simulink model "Environment"  (R2024a)
settings: Solver=ode15s  StartTime=0.0  StopTime=50  FixedStep=0.04  MaxStep=0.04  RelTol=1e-3
values from neighbouring files (symbols this model uses):
  h = 2.7    [Variabili.m]
  traiettoria = [x', y']    [generatoreTraiettoria.m]    (also in generatoreTraiettoria2.m; tra3.m)
  w = 1.4    [Variabili.m]
libraries: simulink x2, rllib x1
settings Model: Creator=Luzi  LastModifiedBy=francesco
settings RTWCC: GPUComputeCapability=3.5

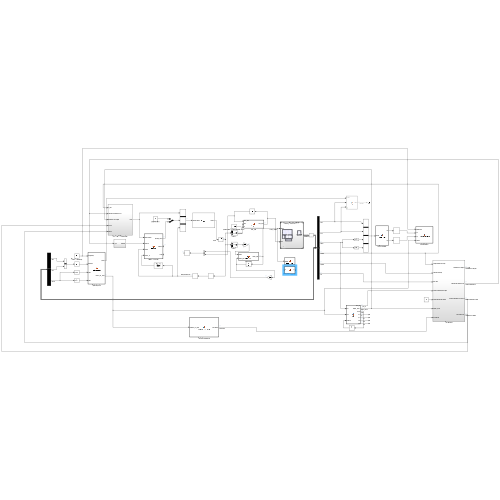
[thumbnail: Simulink's stored preview of the top-level diagram]
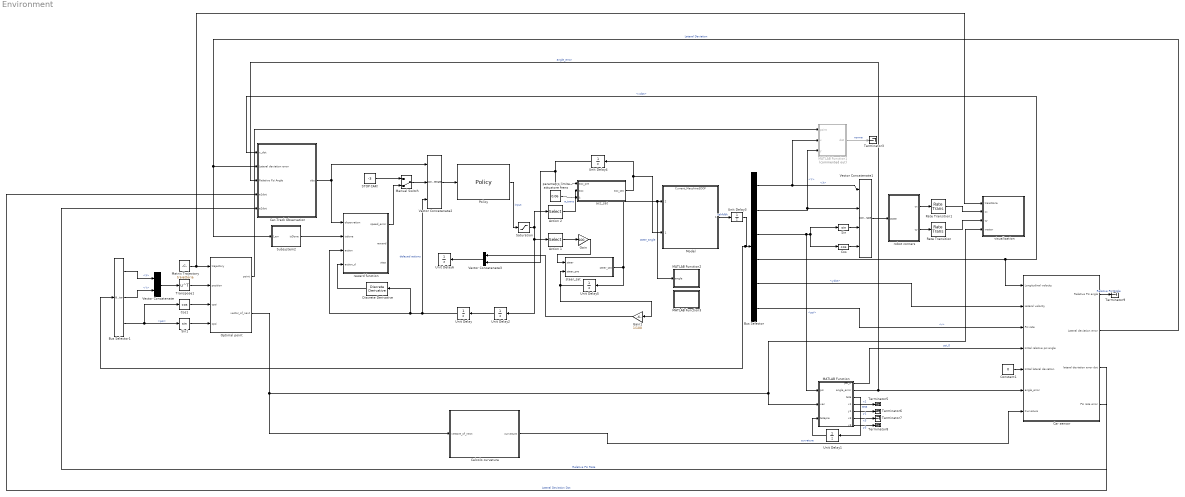
== system Environment ==
  Action 1 : Selector  InputPortWidth=2  IndexOptions=Index vector (dialog)  Indices=1  OutputSizes=1
  Action 2 : Selector  InputPortWidth=2  IndexOptions=Index vector (dialog)  Indices=2  OutputSizes=1
  Bus Selector : BusSelector  OutputSignals=InertFrm.Cg.Disp.X,InertFrm.Cg.Disp.Y,InertFrm.Cg.Ang.psi,BdyFrm.Cg.Vel.xdot,BdyFrm.Cg.Vel.ydot,BdyFrm.Cg.AngVel.r
  Bus Selector1 : BusSelector  OutputSignals=InertFrm.Cg.Disp.X,InertFrm.Cg.Disp.Y,InertFrm.Cg.Ang.psi
  Calcolo curvatura : MATLAB Function  TreatAsAtomicUnit=on
  Car sensor : Subsystem
  Car-Track Observation : Subsystem
  Constant1 : Constant  Value=0
  Cos : Trigonometry  Operator=cos
  Cos1 : Trigonometry  Operator=cos
  Discrete Derivative : simulink/Discrete/Discrete Derivative  gainval=0.1  ICPrevScaledInput=0.0  OutMin=[]  OutMax=[]  OutDataType=fixdt(1, 16)  OutScaling=2^-10  DoSatur=off
  Gain : Gain  Gain=100
  Gain1 : Gain  Gain=1/100
  MATLAB Function : MATLAB Function  TreatAsAtomicUnit=on
  MATLAB Function1 : MATLAB Function  Commented=on  TreatAsAtomicUnit=on
  MATLAB Function2 : MATLAB Function  TreatAsAtomicUnit=on
  MATLAB Function3 : MATLAB Function  TreatAsAtomicUnit=on
  Manual Switch : ManualSwitch  CurrentSetting=0
  Matrix Trajectory : Constant  Value=traiettoria  SampleTime=60
  Model : ModelReference  ModelNameDialog=Current_Macchina3DOF.slx  SimulationMode=Normal  ModelReferenceVersion=1.72
      settings: PortSchema="{\"entries\":[{\"content\":{\"sides\":[{\"content\":{\"connectorIds\":[\"In2\",\"In1\"]},\"type\":\"ConnectorPlacement.EquallySpacedRectSide\",\"uuid\":\"b5a44853-6584-4a50-847d-9a0b1c5ea9ac\"},{\"content\":{\"connectorIds\":[\"Out1\"],\"side\":\"RIGHT\"},\"type\":\"ConnectorPlacement.EquallySpacedRectSide\",\"uuid\":\"bfcb6c88-1d93-4f70-bf16-2c719fa247ba\"},{\"content\":{\"side\":\"TOP\"},\"type\":\"ConnectorPlacement.EquallySpacedRectSide\",\"uuid\":\"3385b00b-6ed4-40a5-8204-01acdd431cf5\"}]},\"type\":\"ConnectorPlacement.EquallySpacedConnector\",\"uuid\":\"3bb36942-6fbc-4d27-a33b-ca1de48b267b\"}],\"packageUris\":[\"http://schema.mathworks.com/mf0/Connector/R2020b\"],\"version\":\"1.0\"}"
  Optimal point : MATLAB Function  TreatAsAtomicUnit=on
  Policy : rllib/Policy  MATFile=/Users/francesco/Repository/FS/HL/High Level Control RL_Training/agentData25hz.mat  PolicyParamsAsInput=off  PolicyParamsBusName=policy_param_bus  SimUsingCodegen=off
  Rate Transition : RateTransition
  Rate Transition1 : RateTransition
  STOP CAR! : Constant  Value=-3
  Saturation : Saturate  UpperLimit=1  LowerLimit=-1
  Sin : Trigonometry
  Sin1 : Trigonometry
  Subsystem2 : Subsystem
  Terminator{3,5..9} (6 alike) : Terminator
  Transpose1 : Math  Operator=transpose
  Unit Delay{,1..6} (7 alike) : UnitDelay  SampleTime=-1  HasFrameUpgradeWarning=on
  Vector Concatenate : Concatenate
  Vector Concatenate1 : Concatenate  NumInputs=4
  Vector Concatenate2 : Concatenate  NumInputs=3
  Vector Concatenate3 : Concatenate
  acc_sat : MATLAB Function  TreatAsAtomicUnit=on
  parametro limite attuatore freno : Constant  Value=0.06
  reward function : MATLAB Function  TreatAsAtomicUnit=on
  robot corners : MATLAB Function  TreatAsAtomicUnit=on
  steer_sat : MATLAB Function  TreatAsAtomicUnit=on
  visualization : MATLAB Function  TreatAsAtomicUnit=on
  wires:
  Policy/1 -> Saturation/1  "input"
  Bus Selector/6 -> Car sensor/3(Psi rate)  "<r>"
  Bus Selector/4 -> Car sensor/1(Longitudinal velocity), Car-Track Observation/1(x_dot)  "<xdot>"
  Sin/1 -> Vector Concatenate1/3
  Cos/1 -> Vector Concatenate1/4
  Unit Delay2/1 -> Unit Delay/1
  Bus Selector1/1 -> Vector Concatenate/1  "<X>"
  Bus Selector1/2 -> Vector Concatenate/2  "<Y>"
  Matrix Trajectory/1 -> Optimal point/1(trajectory), visualization/1(traiettoria)
  Cos1/1 -> Optimal point/3(cpsi)
  Vector Concatenate/1 -> Transpose1/1
  Transpose1/1 -> Optimal point/2(position)
  robot corners/2(cy) -> Rate Transition/1
  robot corners/1(cx) -> Rate Transition1/1
  Unit Delay3/1 -> Bus Selector1/1, Bus Selector/1
  Bus Selector1/3 -> Cos1/1, Sin1/1  "<psi>"
  Sin1/1 -> Optimal point/4(spsi)
  Vector Concatenate1/1 -> robot corners/1(state)
  Bus Selector/5 -> Car sensor/2(Lateral velocity)  "<ydot>"
  Calcolo curvatura/1(curvatura) -> Car sensor/7(Curvature)  "curvature"
  MATLAB Function/1(psi_0) -> Car sensor/4(Initial relative psi angle)  "psi_0"
  Car sensor/3(lateral deviation error dot) -> Car-Track Observation/4(e1dot)  "Lateral Deviation Dot"
  Car sensor/4(Psi rate error) -> Car-Track Observation/5(e2dot)  "Relative Psi Rate"
  Car sensor/2(Lateral deviation error) -> Car-Track Observation/2(Lateral deviation error), Subsystem2/1(l_err)  "Lateral Deviation"
  Vector Concatenate2/1 -> Policy/1
  Car-Track Observation/1(obs) -> Vector Concatenate2/1, reward function/1(observation)
  Optimal point/1(point) -> MATLAB Function1/1(point)
  Optimal point/2(vector_of_next) -> Calcolo curvatura/1(vettore_of_next), visualization/4(vector), MATLAB Function/2(vec)
  Model/1 -> Unit Delay3/1  "vehfdbk"
  Rate Transition1/1 -> visualization/2(cx)
  Rate Transition/1 -> visualization/3(cy)
  Unit Delay/1 -> Vector Concatenate2/3, reward function/3(action), Discrete Derivative/1  "delayed actions"
  Saturation/1 -> Unit Delay2/1, Action 1/1, Action 2/1
  Discrete Derivative/1 -> reward function/4(action_d)
  Bus Selector/1 -> Vector Concatenate1/1, MATLAB Function1/2(x)  "<X>"
  Bus Selector/2 -> MATLAB Function1/3(y), Vector Concatenate1/2  "<Y>"
  Bus Selector/3 -> MATLAB Function/1(psi), Cos/1, Sin/1  "<psi>"
  MATLAB Function/2(angle_error) -> Car-Track Observation/3(Relative Psi Angle), Car sensor/6(angle_error)  "angle_error"
  MATLAB Function1/1(dist) -> Terminator3/1  "norma"
  MATLAB Function/3(teta) -> Unit Delay1/1  "teta"
  Constant1/1 -> Car sensor/5(Initial lateral deviation)
  MATLAB Function/4(x1) -> Terminator5/1  "x1"
  MATLAB Function/5(y1) -> Terminator6/1  "y1"
  MATLAB Function/6(x3) -> Terminator7/1  "x3"
  MATLAB Function/7(y3) -> Terminator8/1  "y3"
  Car sensor/1(Relative Psi angle) -> Terminator9/1  "Relative Psi Angle"
  Unit Delay1/1 -> MATLAB Function/3(tetapre)
  Unit Delay4/1 -> Vector Concatenate3/2, acc_sat/1(acc_pre)
  acc_sat/1(acc_sat) -> Unit Delay4/1, Model/1
  Unit Delay5/1 -> steer_sat/2(steer_pre), Gain1/1
  steer_sat/1(steer_sat) -> Unit Delay5/1, MATLAB Function2/1(angle), Model/2  "steer_angle"
  Action 1/1 -> Gain/1
  Subsystem2/1(isDone) -> reward function/2(isdone)
  Gain/1 -> steer_sat/1(steer)
  Vector Concatenate3/1 -> Unit Delay6/1
  Gain1/1 -> Vector Concatenate3/1
  reward function/1(speed_error) -> Manual Switch/2
  Manual Switch/1 -> Vector Concatenate2/2
  STOP CAR!/1 -> Manual Switch/1
  Action 2/1 -> acc_sat/2(acc)  "a_trans"
  parametro limite attuatore freno/1 -> acc_sat/3(k)

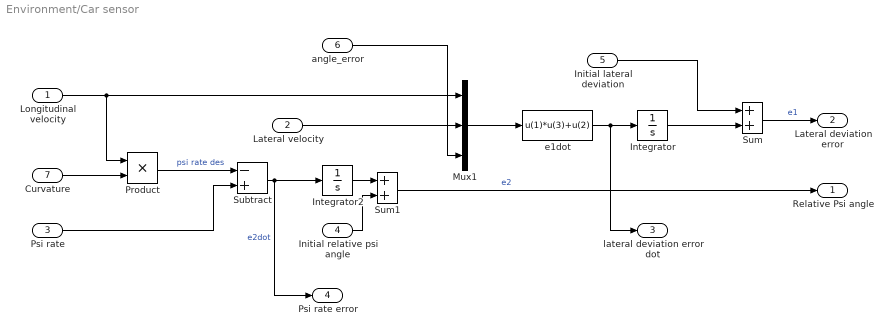
== system Environment/Car sensor ==
  Longitudinal velocity : Inport
  Lateral velocity : Inport  Port=2
  Psi rate : Inport  Port=3
  Initial relative psi angle : Inport  Port=4
  Initial lateral deviation : Inport  Port=5
  angle_error : Inport  Port=6
  Curvature : Inport  Port=7
  Integrator : Integrator
  Integrator2 : Integrator
  Mux1 : Mux  Inputs=[1 1 1]
  Product : Product
  Subtract : Sum  Inputs=-+
  Sum : Sum
  Sum1 : Sum
  e1dot : Fcn  Expr=u(1)*u(3)+u(2)
  Relative Psi angle : Outport  VectorParamsAs1DForOutWhenUnconnected=off
  Lateral deviation error : Outport  Port=2  VectorParamsAs1DForOutWhenUnconnected=off
  lateral deviation error dot : Outport  Port=3  VectorParamsAs1DForOutWhenUnconnected=off
  Psi rate error : Outport  Port=4  VectorParamsAs1DForOutWhenUnconnected=off
  wires:
  Curvature/1 -> Product/2
  Sum1/1 -> Relative Psi angle/1  "e2"
  Mux1/1 -> e1dot/1
  Initial lateral deviation/1 -> Sum/1
  e1dot/1 -> lateral deviation error dot/1, Integrator/1
  Integrator/1 -> Sum/2
  Longitudinal velocity/1 -> Product/1, Mux1/1
  Lateral velocity/1 -> Mux1/2
  Sum/1 -> Lateral deviation error/1  "e1"
  Integrator2/1 -> Sum1/1
  Initial relative psi angle/1 -> Sum1/2
  Product/1 -> Subtract/1  "psi rate des"
  Psi rate/1 -> Subtract/2
  Subtract/1 -> Psi rate error/1, Integrator2/1  "e2dot"
  angle_error/1 -> Mux1/3

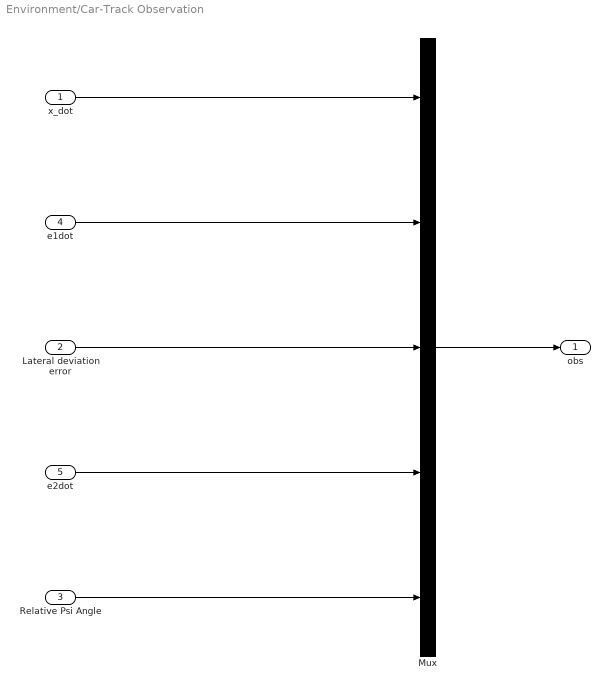
== system Environment/Car-Track Observation ==
  x_dot : Inport
  Lateral deviation error : Inport  Port=2
  Relative Psi Angle : Inport  Port=3
  e1dot : Inport  Port=4
  e2dot : Inport  Port=5
  Mux : Mux  Inputs=5
  obs : Outport  VectorParamsAs1DForOutWhenUnconnected=off
  wires:
  Lateral deviation error/1 -> Mux/3
  Relative Psi Angle/1 -> Mux/5
  Mux/1 -> obs/1
  x_dot/1 -> Mux/1
  e1dot/1 -> Mux/2
  e2dot/1 -> Mux/4

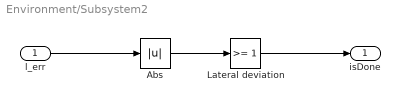
== system Environment/Subsystem2 ==
  l_err : Inport
  Abs : Abs  SaturateOnIntegerOverflow=off
  Lateral deviation : simulink/Logic and Bit Operations/Compare To Constant  relop=>=  const=1  OutDataTypeStr=boolean
  isDone : Outport  VectorParamsAs1DForOutWhenUnconnected=off
  wires:
  Abs/1 -> Lateral deviation/1
  l_err/1 -> Abs/1
  Lateral deviation/1 -> isDone/1

== matlab function Environment/MATLAB Function1 ==
  data: point input; x input; y input; dist output
function dist = fcn(point,x,y)

dist=sqrt((point(1)-x)^2+(point(2)-y)^2);

end

== matlab function Environment/Calcolo curvatura ==
  data: vettore_of_next input; curvatura output
function curvatura = calcola_curvatura(vettore_of_next)
    % Input:
    %   vettore_of_next: 3x2 matrix containing three points on the curve
    % Output:
    %   curvatura: vector containing the calculated curvature values

    % Extract x and y coordinates from the curve points
    x = vettore_of_next(:, 1);
    y = vettore_of_next(:, 2);

    % Calculate the first derivatives of x and y
    dx = diff(x);
    dy = diff(y);

    % Calculate the second derivatives of x and y
    d2x = diff(dx);
    d2y = diff(dy);

    % Calculate curvature using the formula: curvature = (dx * d2y - dy * d2x) / (dx^2 + dy^2)^(3/2)
    numeratore = dx(2:end) .* d2y - dy(2:end) .* d2x;
    denominatore = (dx(2:end).^2 + dy(2:end).^2).^(3/2);
    curvatura = numeratore ./ denominatore;

    % Handle any NaN values by setting them to zero
    for i = 1:length(curvatura)
        if (isnan(curvatura(i)))
            curvatura(i) = 0;
        end
    end
end

== matlab function Environment/steer_sat ==
  data: steer input; steer_sat output; steer_pre input
function steer_sat = Sat_steer(steer,steer_pre)
    steer_sat=steer;
    if(steer-steer_pre>5)
        steer_sat=steer_pre+5;
    elseif(steer-steer_pre<-5)
        steer_sat=steer_pre-5;

    end
end

== matlab function Environment/acc_sat ==
  data: acc_pre input; acc_sat output; acc input; k input
function acc_sat = Sat_acc(acc_pre,acc,k)
    if(acc<0 && acc_pre<=0)
        acc_sat=acc;
        if(acc-acc_pre>k)
            acc_sat=acc_pre+k;
        elseif (acc-acc_pre<-k)
            acc_sat=acc_pre-k;
        end

    elseif(acc<0 && acc_pre>0)
        acc_sat=acc;
        if(acc-acc_pre>k)
           acc_sat=0;
        elseif (acc-acc_pre<-k)
            acc_sat=0;        
        end

    elseif(acc>=0 && acc_pre<0)
        acc_sat=acc;
        if(abs(acc_pre)>k)          
            if(acc-acc_pre>k)
               acc_sat=acc_pre+k;
            elseif (acc-acc_pre<-k)
                acc_sat=acc_pre+k;        
            end
        else
            acc_sat=0;
        end        
    
    else
        acc_sat=acc;
    end

end

== matlab function Environment/MATLAB Function2 ==
  data: angle input
function sendSerial(angle)
%#codegen
coder.extrinsic('manageSerial');

% Open the serial port if not already opened
manageSerial(0, 'open');

% Send the angle data
manageSerial(angle, 'write');

== matlab function Environment/MATLAB Function3 ==
function closeSerial()
%#codegen
coder.extrinsic('manageSerial');

% Close the serial port
manageSerial(0, 'close');

== matlab function Environment/MATLAB Function ==
  data: psi_0 output; psi input; vec input; angle_error output; teta output; x1 output; y1 output; x3 output; y3 output; tetapre input
function [psi_0,angle_error,teta,x1,y1,x3,y3] = fcn(psi,vec,tetapre)
    x1=vec(1,1);
    y1=vec(1,2);
    x3=vec(3,1);
    y3=vec(3,2);
    teta=atan2((y3-y1),(x3-x1));


     if(abs(tetapre-teta)>pi/4 && abs(tetapre-teta)<1.1*pi)%ATTENZIONE: PROVVISORIO PER RISOLVERE IL PROBLEMA DELL'INCROCIO
         teta=tetapre;
     end



    angle_error=psi-teta;
    if angle_error>pi
        angle_error=angle_error-2*pi;
    elseif angle_error<-pi
        angle_error=angle_error+2*pi;
    end
    persistent initialValue
    if isempty(initialValue)
        initialValue = angle_error; 
    end
    psi_0 = initialValue;
end

== matlab function Environment/reward function ==
  data: speed_error output; observation input; isdone input; action input; action_d input; reward output; stop output
function [speed_error, reward, stop] = reward(observation, isdone, action, action_d)
    % Input:
    %   observation: vector containing relevant state information
    %   isdone: flag indicating whether the episode is finished
    %   action: vector representing the action taken
    %   action_d: vector representing the action derivatives
    % Output:
    %   speed_error: computed speed error based on the current velocity
    %   reward: calculated reward value considering various factors
    %   stop: flag indicating whether the episode should stop

    v = observation(1); % observed velocity
    e1 = observation(3); % lateral deviation
    e2 = observation(5); % relative psi angle error
    bonus_pos = 0;
    % bonusr = 0;

    % Calculate speed error based on the current velocity
    speed_error = 3 * (v - 3)^2 / ((v - 3)^2 + 2); % 3m/s
    %speed_error = 8 * (v - 9)^2 / ((v - 15)^2 + 1); MAX
    s_dot = action_d(1);
    a_dot = action_d(2);
    steer = action(1);
    a_trans = action(2);

    % Apply bonus based on lateral deviation
    
    if (e1^2 < 0.04)
        bonus_pos = 2;
    end

    if (e1^2 < 0.01)
        bonus_pos = bonus_pos + 0.5;
    end

    % Calculate the reward value
    reward = -(2 * e1^2 + 0.5*e2^2) - 50 * isdone + bonus_pos - speed_error - 0.25 * a_dot^2 - 1 * s_dot^2;
    % aumentare penalità sulle derivate e diminuire leggermente quella
    % sull'errore d'angolo magari passare a 0.25, forse diminuire il bonus
    % di deviazione laterale
    stop = isdone;
end

%funzione countorf(x,y,z) per mappatura ricompenra e colorbar da inserire
%(nel editor matlab) per il controllo funzionalità

== matlab function Environment/Optimal point ==
  data: trajectory input; point output; position input; cpsi input; spsi input; vector_of_next output
function [point, vector_of_next] = optimalpoint(trajectory, position, cpsi, spsi)
    % Input:
    %   trajectory: Nx2 matrix representing the trajectory points
    %   position: 1x2 row vector representing the current position (xy)
    %   cpsi, spsi: components of the velocity direction
    % Output:
    %   point: 1x2 row vector representing the optimal point on the trajectory
    %   vector_of_next: 3x2 matrix containing the optimal point and the next two points

    % Initialize the matrix for the next points
    vector_of_next = zeros(3, 2);

    % Calculate distances between the current position and points on the trajectory
    N = size(trajectory, 1);
    distanceVector = zeros(N, 2);
    distanceValue = zeros(N, 1);

    for i = 1:N
        distanceVector(i, :) = trajectory(i, :) - position;
        distanceValue(i) = sqrt(distanceVector(i, 1)^2 + distanceVector(i, 2)^2);
    end

    % Find indices of the three nearest points
    [~, indx] = mink(distanceValue, 3);

    % Normalize distances and velocity direction
    distance1norm = distanceVector(indx(1), :) / norm(distanceVector(indx(1), :));
    distance2norm = distanceVector(indx(2), :) / norm(distanceVector(indx(2), :));
    distance3norm = distanceVector(indx(3), :) / norm(distanceVector(indx(3), :));
    direction = [cpsi, spsi];
    velocitynorm = direction;

    % Calculate dot product between normalized distances and velocity direction
    dotmatrix = [dot(distance1norm, velocitynorm), dot(distance2norm, velocitynorm), dot(distance3norm, velocitynorm)];

    % Find the index of the maximum dot product
    [~, I] = max(dotmatrix);

    % Get the optimal point
    point = trajectory(indx(I), :);

    if(indx(I)==1)
        vector_of_next(1,:)=point;
    else   
        vector_of_next(1,:)=trajectory(indx(I)-1,:);
    end

    vector_of_next(2,:)=point;

    if(indx(I)==length(trajectory))
        vector_of_next(3,:)=point;
    else
        vector_of_next(3,:)=trajectory(indx(I)+1,:);
    end
end

== matlab function Environment/robot corners ==
  data: state input; cx output; cy output; h parameter; w parameter
function [cx,cy] = getcorners(state,h,w)

    % preallocate outputs
    % cx = zeros(4,1);
    % cy = zeros(4,1);
    
    % extract individual components
    x = state(1);
    y = state(2);
    s = state(3);
    c = state(4);
    
    % four corners
    p = [h,-h,-h,h;w,w,-w,-w]/2;
    
    % rotation matrix
    M = [c,-s;s,c];
    
    % rotate points
    p = M*p;
    % translate and extract x,y
    cx = x*ones(1,4) + p(1,:);
    cy = y*ones(1,4) + p(2,:);

end

== matlab function Environment/visualization ==
  data: traiettoria input; cx input; cy input; vector input
function drawEnvironment(traiettoria,cx,cy,vector)
point=vector(end,:);
coder.extrinsic("plotRobot");
plotRobot(cx,cy,point,traiettoria);
